simulink model "TanqueComp"  (R2020a)
settings: Solver=VariableStepAuto  StartTime=0.0  StopTime=20  RelTol=1e-3
undefined symbols (not defined in the file or in its folder): A, B, C, D, eFinal, eInicial, h0
settings Model: Creator=a1  LastModifiedBy=a1

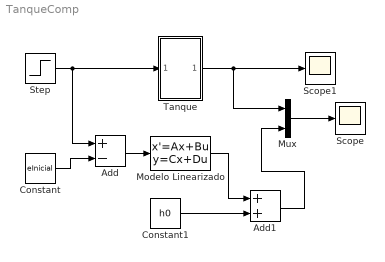
== system TanqueComp ==
  Add : Sum  Inputs=+-
  Add1 : Sum
  Constant : Constant  Value=eInicial
  Constant1 : Constant  Value=h0
  Modelo Linearizado : StateSpace  A=A  B=B  C=C  D=D  InitialCondition=0
  Mux : Mux  Inputs=2
  Scope : Scope
  Scope1 : Scope
  Step : Step  Before=eInicial  After=eFinal  SampleTime=0
  Tanque : Subsystem
  wires:
  Tanque/1(h(t)) -> Scope1/1, Mux/1
  Mux/1 -> Scope/1
  Step/1 -> Add/1, Tanque/1(e(t))
  Add/1 -> Modelo Linearizado/1
  Constant/1 -> Add/2
  Modelo Linearizado/1 -> Add1/1
  Add1/1 -> Mux/2
  Constant1/1 -> Add1/2

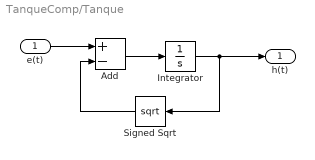
== system TanqueComp/Tanque ==
  e(t) : Inport
  Add : Sum  Inputs=+-
  Integrator : Integrator  InitialCondition=h0
  Signed Sqrt : Sqrt  OutputSignalType=real  SaturateOnIntegerOverflow=on
  h(t) : Outport
  wires:
  e(t)/1 -> Add/1
  Signed Sqrt/1 -> Add/2
  Add/1 -> Integrator/1
  Integrator/1 -> h(t)/1, Signed Sqrt/1
